simulink library "commanabbnd2"  (Simulink 5.0)
values from neighbouring files (symbols this model uses):
  i = i + 1    (= 3)    [eyediasi2.m]
undefined symbols (not defined in the file or in its folder): den, num
libraries: dspsigattribs x20, commanabbnd2 x3, comminteg2 x3
settings Model: RequirementInfo=9  CovMetricSettings=d  Creator=tdelve  LastModifiedBy=mmclerno

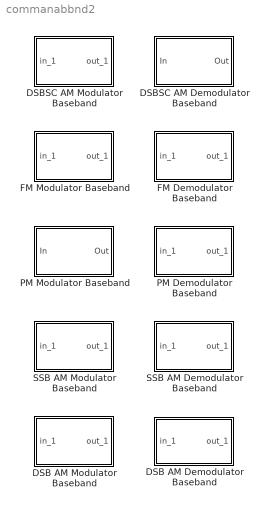
== system commanabbnd2 ==
  DSB AM Demodulator Baseband : Subsystem  mask(DSB AM Demodulator Baseband){Offset=1, num=[4.57 9.14 4.57]*.01, den=[1 -1.3108 .4936], Ph=0, ts=0.001}
      mask prompts: Offset "Output signal offset:"; num "Lowpass filter numerator:"; den "Lowpass filter denominator:"; Ph "Initial phase (rad):"; ts "Sample time (s):"
      mask help: Demodulate the complex envelope of a double-sideband amplitude modulated signal. The input signal must be a sample-based scalar.The output is a 1-D scalar.
      mask init:
      | if ((length(Ph)~=1) | (length(Offset)~=1) | (length(ts)~=1))error('Mask parameters must be scalar values.');end;
      mask Help: helpview(commbhelp)
      mask Display:
      | plot(0,0,100,100,[5+4.5*[0:.15:10] 50 50 50 50+4.5*[0:10]],[85+10*[sin([0:.15:10]*pi*2+cumsum(sin([0:.15:10]*pi/5))/2)] 85 99 75   10*sin([0:10]*pi/5)+85]);
      | disp('DSB AM')
  DSB AM Modulator Baseband : Subsystem  mask(DSB AM Modulator Baseband){Offset=1, Ph=0}
      mask prompts: Offset "Input signal offset:"; Ph "Initial phase (rad):"
      mask help: Output complex envelope of a double-sideband amplitude modulated signal. The input signal must be a sample-based scalar. The output is a 1-D scalar.
      mask init:
      | if ((length(Ph)~=1) | (length(Offset)~=1))error('Mask parameters must be scalar values.');end;
      mask Help: helpview(commbhelp)
      mask Display:
      | plot(0,0,100,100,[4.5*[0:10]+5 50 50 50 50+4.5*[0:.15:10]],[10*sin([0:10]*pi/5)+85 85 99 75 85+10*[sin([0:.15:10]*pi*2+cumsum(sin([0:.15:10]*pi/5))/2)]]);
      | disp('DSB AM')
  DSBSC AM Demodulator Baseband : Subsystem  mask(DSBSC AM Demodulator Baseband){num=[4.57 9.14 4.57]*.01, den=[1 -1.3108 .4936], Ph=pi/2, ts=0.001}
      mask prompts: num "Lowpass filter numerator:"; den "Lowpass filter denominator:"; Ph "Initial phase (rad):"; ts "Sample time (s):"
      mask help: Demodulate the complex envelope of a double-sideband suppressed carrier amplitude modulated signal. The input signal must be a sample-based scalar. The output is a 1-D scalar.
      mask init:
      | if ((length(Ph)~=1) | (length(ts)~=1))error('Mask parameters must be scalar values.');end;
      | pi2=pi*2;
      mask Help: helpview(commbhelp)
      mask Display:
      | plot(0,0,100,100,[5+4.5*[0:.15:10] 50 50 50 50+4.5*[0:10]],[85+10*[sin([0:.15:10]*pi*2+cumsum(sin([0:.15:10]*pi/5))/2)] 85 99 75   10*sin([0:10]*pi/5)+85]);
      | disp('DSBSC AM')
  DSBSC AM Modulator Baseband : Subsystem  mask(DSBSC AM Modulator Baseband){Ph=pi/2}
      mask prompts: Ph "Initial phase (rad):"
      mask help: Output the complex envelope of a double-sideband suppressed carrier amplitude modulated signal. The input signal must be a sample-based scalar. The output is a 1-D scalar.
      mask init:
      | if (length(Ph)~=1) error('Mask parameters must be scalar values.');end;
      | x1=cos(Ph);x2=sin(Ph);pi2=2*pi;
      mask Help: helpview(commbhelp)
      mask Display:
      | plot(0,0,100,100,[4.5*[0:10]+5 50 50 50 50+4.5*[0:.15:10]],[10*sin([0:10]*pi/5)+85 85 99 75 85+10*[sin([0:.15:10]*pi*2+cumsum(sin([0:.15:10]*pi/5))/2)]]);
      | disp('DSBSC AM')
  FM Demodulator Baseband : Subsystem  mask(FM Demodulator Baseband){Ph=0, HzPerVolt=1, num=[4.57 9.14 4.57]*.01, den=[1 -1.3108 .4936], ts=0.001}
      mask prompts: Ph "Initial phase (rad):"; HzPerVolt "Modulation constant (Hertz per volt):"; num "Lowpass filter numerator:"; den "Lowpass filter denominator:"; ts "Sample time (s):"
      mask help: Demodulate the complex envelope of a frequency-modulated signal. The input signal must be a sample-based scalar. The output is a 1-D scalar.
      mask init:
      | if ((length(Ph)~=1) | (length(HzPerVolt)~=1) | (length(ts)~=1))error('Mask parameters must be scalar values.');end;
      | pi2=2*pi;
      | Kc=2*pi*HzPerVolt;
      mask Help: helpview(commbhelp)
      mask Display:
      | plot(0,0,100,100,[5+4.5*[0:.15:10] 50 50 50 50+4.5*[0:10]],[85+10*[sin([0:.15:10]*pi*2+cumsum(sin([0:.15:10]*pi/5))/2)] 85 99 75   10*sin([0:10]*pi/5)+85]);
      | disp('FM')
  FM Modulator Baseband : Subsystem  mask(FM Modulator Baseband){Ph=0, HzPerV=1, ts=0.001, td=Inf}
      mask prompts: Ph "Initial phase (rad):"; HzPerV "Modulation constant (Hertz per volt):"; ts "Sample time (s):"; td "Symbol interval (s):"
      mask help: Output complex baseband signal frequency-modulated by the input signal. For digital modulation, set the Symbol Interval parameter to the desired symbol. For analog modulation, set the Symbol Interval parameter to Inf. The input signal must be a sample-based scalar. The output is a 1-D scalar.
      mask init:
      | if ((length(Ph)~=1) | (length(HzPerV)~=1) | (length(ts)~=1) | (length(td)~=1))error('Mask parameters must be scalar values.');end;
      | Kc =2*pi*HzPerV;if isinf(td),td=realmax;end;
      mask Help: helpview(commbhelp)
      mask Display:
      | plot(0,0,100,100,[4.5*[0:10]+5 50 50 50 50+4.5*[0:.15:10]],[10*sin([0:10]*pi/5)+85 85 99 75 85+10*[sin([0:.15:10]*pi*2+cumsum(sin([0:.15:10]*pi/5))/2)]]);
      | disp('FM')
  PM Demodulator Baseband : Subsystem  mask(PM Demodulator Baseband){Ph=0, Kc=1, num=[4.57 9.14 4.57]*.01, den=[1 -1.3108 .4936], HzPerVolt=1, ts=0.001}
      mask prompts: Ph "Initial phase (rad):"; Kc "Modulation constant (Radians per volt):"; num "Lowpass filter numerator:"; den "Lowpass filter denominator:"; HzPerVolt "VCO gain (Hertz per volt):"; ts "Sample time (s):"
      mask help: Demodulate the complex envelope of a phase-modulated signal. The input signal must be a sample-based scalar. The output is a 1-D scalar.
      mask init:
      | if ((length(Ph)~=1) | (length(HzPerVolt)~=1) | (length(ts)~=1) | (length(Kc)~=1))error('Mask parameters must be scalar values.');end;
      | Kv=2*pi*HzPerVolt;
      mask Help: helpview(commbhelp)
      mask Display:
      | plot(0,0,100,100,[5+4.5*[0:.15:10] 50 50 50 50+4.5*[0:10]],[85+10*[sin([0:.15:10]*pi*2+cumsum(sin([0:.15:10]*pi/5))/2)] 85 99 75   10*sin([0:10]*pi/5)+85]);
      | disp('PM')
  PM Modulator Baseband : Subsystem  mask(PM Modulator Baseband){Ph=0, Kc=1}
      mask prompts: Ph "Initial phase (rad):"; Kc "Modulation constant (Radians per volt):"
      mask help: Output the complex envelope of a phase-modulated signal. The input signal must be a sample-based scalar. The output is a 1-D scalar.
      mask init:
      | if ((length(Ph)~=1) | (length(Kc)~=1))error('Mask parameters must be scalar values.');end;
      mask Help: helpview(commbhelp)
      mask Display:
      | plot(0,0,100,100,[4.5*[0:10]+5 50 50 50 50+4.5*[0:.15:10]],[10*sin([0:10]*pi/5)+85 85 99 75 85+10*[sin([0:.15:10]*pi*2+cumsum(sin([0:.15:10]*pi/5))/2)]]);
      | disp('PM')
  SSB AM Demodulator Baseband : Subsystem  mask(SSB AM Demodulator Baseband){num=[4.57 9.14 4.57]*.01, den=[1 -1.3108 .4936], Ph=0, ts=0.001}
      mask prompts: num "Lowpass filter numerator:"; den "Lowpass filter denominator:"; Ph "Initial phase (rad):"; ts "Sample time (s):"
      mask help: Demodulate the complex envelope of a single-sideband amplitude modulated signal. The input signal must be a sample-based scalar. The output is a 1-D scalar.
      mask init:
      | if ((length(Ph)~=1) | (length(ts)~=1))error('Mask parameters must be scalar values.');end;
      | x1=cos(-Ph);x2=sin(-Ph);
      mask Help: helpview(commbhelp)
      mask Display:
      | plot(0,0,100,100,[5+4.5*[0:.15:10] 50 50 50 50+4.5*[0:10]],[85+10*[sin([0:.15:10]*pi*2+cumsum(sin([0:.15:10]*pi/5))/2)] 85 99 75   10*sin([0:10]*pi/5)+85]);
      | disp('SSB AM')
  SSB AM Modulator Baseband : Subsystem  mask(SSB AM Modulator Baseband){Ph=0, ban=10, dly=0.01, ts=0.001, sd=upper}
      mask prompts: Ph "Initial phase (rad):"; ban "Bandwidth of the input signal (Hz):"; dly "Time delay for Hilbert transform filter (s):"; ts "Sample time (s):"; sd "Sideband to modulate:"
      mask help: Output complex envelope of a single-sideband amplitude modulated signal. The input signal must be a sample-based scalar. The output is a 1-D scalar.
      mask init:
      | if ((length(Ph)~=1) | (length(ban)~=1) | (length(ts)~=1) | (length(dly)~=1))error('Mask parameters must be scalar values.');end;
      | if dly/ts<3 error('Time delay is too small compared to the Sample time value');end;
      | if ban>1/ts, ban=1/ts-ts;end;if(dly/ts>1000)
      | error(['The filter coefficients will take too long to compute.'...
      |         'Try reducing the length of the impulse response by increasing the sample time, or decreasing the delay'])
      | else
      | [num,den]=hilbiir(ts,dly,ban);pi2=2*pi;pih=pi/2;
      | k=-1;if lower(sd)=='lower',k=1;end;
      | end;
      mask Help: helpview(commbhelp)
      mask StyleString: edit,edit,edit,edit,popup(Upper|Lower)
      mask Display:
      | plot(0,0,100,100,[4.5*[0:10]+5 50 50 50 50+4.5*[0:.15:10]],[10*sin([0:10]*pi/5)+85 85 99 75 85+10*[sin([0:.15:10]*pi*2+cumsum(sin([0:.15:10]*pi/5))/2)]]);
      | disp('SSB AM')

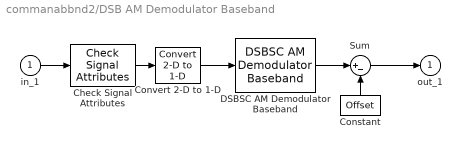
== system commanabbnd2/DSB AM Demodulator Baseband ==
  in_1 : Inport
  Check Signal Attributes : dspsigattribs/Check Signal Attributes  SigAttribCheckMethod=Does not match attributes exactly  Complexity=Ignore  Frame=Sample-based  DimsCheckMethod=Is...  Dimensions=Scalar (1-D or 2-D)  DatatypeCheckMethod=Ignore  DatatypeGeneral=Boolean  DtypeFloatSpecific=Any floating-point  DtypeFixedSpecific=Any fixed-point  DtypeIntSpecific=Any integer  SampleMode=Ignore
  Constant : Constant  Orientation=up  Value=Offset
  Convert 2-D to 1-D : dspsigattribs/Convert 2-D to 1-D
  DSBSC AM Demodulator Baseband : commanabbnd2/DSBSC AM Demodulator Baseband  num=num  den=den  Ph=Ph  ts=ts
  Sum : Sum  Inputs=|+-  SaturateOnIntegerOverflow=on  InputSameDT=on
  out_1 : Outport  InitialOutput=0
  wires:
  DSBSC AM Demodulator Baseband/1 -> Sum/1
  in_1/1 -> Check Signal Attributes/1
  Constant/1 -> Sum/2
  Sum/1 -> out_1/1
  Convert 2-D to 1-D/1 -> DSBSC AM Demodulator Baseband/1
  Check Signal Attributes/1 -> Convert 2-D to 1-D/1

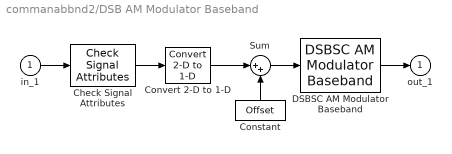
== system commanabbnd2/DSB AM Modulator Baseband ==
  in_1 : Inport
  Check Signal Attributes : dspsigattribs/Check Signal Attributes  SigAttribCheckMethod=Does not match attributes exactly  Complexity=Ignore  Frame=Sample-based  DimsCheckMethod=Is...  Dimensions=Scalar (1-D or 2-D)  DatatypeCheckMethod=Ignore  DatatypeGeneral=Boolean  DtypeFloatSpecific=Any floating-point  DtypeFixedSpecific=Any fixed-point  DtypeIntSpecific=Any integer  SampleMode=Ignore
  Constant : Constant  Orientation=up  Value=Offset
  Convert 2-D to 1-D : dspsigattribs/Convert 2-D to 1-D
  DSBSC AM Modulator Baseband : commanabbnd2/DSBSC AM Modulator Baseband  Ph=Ph
  Sum : Sum  Inputs=|++  SaturateOnIntegerOverflow=on  InputSameDT=on
  out_1 : Outport  InitialOutput=0
  wires:
  Constant/1 -> Sum/2
  in_1/1 -> Check Signal Attributes/1
  Sum/1 -> DSBSC AM Modulator Baseband/1
  DSBSC AM Modulator Baseband/1 -> out_1/1
  Convert 2-D to 1-D/1 -> Sum/1
  Check Signal Attributes/1 -> Convert 2-D to 1-D/1

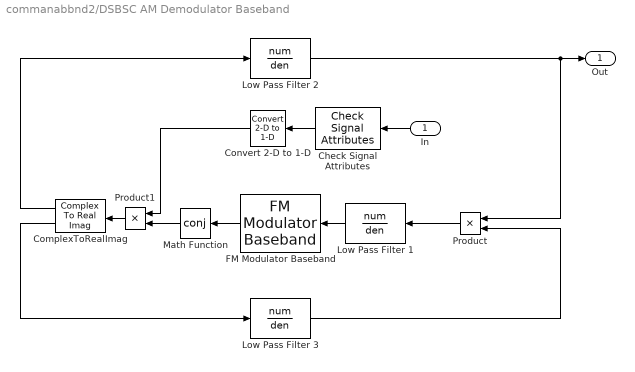
== system commanabbnd2/DSBSC AM Demodulator Baseband ==
  In : Inport  Orientation=left
  Check Signal Attributes : dspsigattribs/Check Signal Attributes  Orientation=left  SigAttribCheckMethod=Does not match attributes exactly  Complexity=Ignore  Frame=Sample-based  DimsCheckMethod=Is...  Dimensions=Scalar (1-D or 2-D)  DatatypeCheckMethod=Ignore  DatatypeGeneral=Boolean  DtypeFloatSpecific=Any floating-point  DtypeFixedSpecific=Any fixed-point  DtypeIntSpecific=Any integer  SampleMode=Ignore
  ComplexToRealImag : ComplexToRealImag  Orientation=left
  Convert 2-D to 1-D : dspsigattribs/Convert 2-D to 1-D  Orientation=left
  FM Modulator Baseband : commanabbnd2/FM Modulator Baseband  Orientation=left  Ph=Ph  HzPerV=1  ts=ts  td=Inf
  Low Pass Filter 1 : DiscreteFilter  Orientation=left  Numerator=num  Denominator=den  SampleTime=ts
  Low Pass Filter 2 : DiscreteFilter  Numerator=num  Denominator=den  SampleTime=ts
  Low Pass Filter 3 : DiscreteFilter  Numerator=num  Denominator=den  SampleTime=ts
  Math Function : Math  Orientation=left  Operator=conj
  Product : Product  Orientation=left  SaturateOnIntegerOverflow=on  InputSameDT=on
  Product1 : Product  Orientation=left  SaturateOnIntegerOverflow=on  InputSameDT=on
  Out : Outport  InitialOutput=0
  wires:
  ComplexToRealImag/1 -> Low Pass Filter 2/1
  ComplexToRealImag/2 -> Low Pass Filter 3/1
  Product/1 -> Low Pass Filter 1/1
  Product1/1 -> ComplexToRealImag/1
  In/1 -> Check Signal Attributes/1
  Math Function/1 -> Product1/2
  FM Modulator Baseband/1 -> Math Function/1
  Low Pass Filter 3/1 -> Product/2
  Low Pass Filter 1/1 -> FM Modulator Baseband/1
  Low Pass Filter 2/1 -> Product/1, Out/1
  Convert 2-D to 1-D/1 -> Product1/1
  Check Signal Attributes/1 -> Convert 2-D to 1-D/1

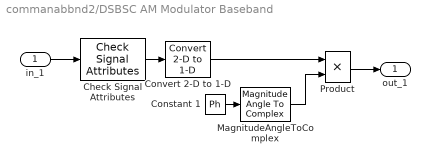
== system commanabbnd2/DSBSC AM Modulator Baseband ==
  in_1 : Inport
  Check Signal Attributes : dspsigattribs/Check Signal Attributes  SigAttribCheckMethod=Does not match attributes exactly  Complexity=Ignore  Frame=Sample-based  DimsCheckMethod=Is...  Dimensions=Scalar (1-D or 2-D)  DatatypeCheckMethod=Ignore  DatatypeGeneral=Boolean  DtypeFloatSpecific=Any floating-point  DtypeFixedSpecific=Any fixed-point  DtypeIntSpecific=Any integer  SampleMode=Ignore
  Constant 1 : Constant  Value=Ph
  Convert 2-D to 1-D : dspsigattribs/Convert 2-D to 1-D
  MagnitudeAngleToComplex : MagnitudeAngleToComplex  Input=Angle  ConstantPart=1
  Product : Product  SaturateOnIntegerOverflow=on  InputSameDT=on
  out_1 : Outport  InitialOutput=0
  wires:
  in_1/1 -> Check Signal Attributes/1
  MagnitudeAngleToComplex/1 -> Product/2
  Constant 1/1 -> MagnitudeAngleToComplex/1
  Product/1 -> out_1/1
  Convert 2-D to 1-D/1 -> Product/1
  Check Signal Attributes/1 -> Convert 2-D to 1-D/1

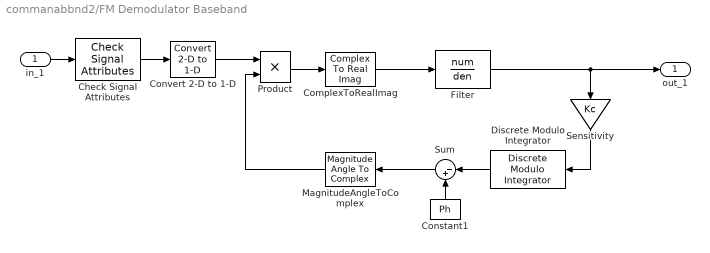
== system commanabbnd2/FM Demodulator Baseband ==
  in_1 : Inport
  Check Signal Attributes : dspsigattribs/Check Signal Attributes  SigAttribCheckMethod=Does not match attributes exactly  Complexity=Ignore  Frame=Sample-based  DimsCheckMethod=Is...  Dimensions=Scalar (1-D or 2-D)  DatatypeCheckMethod=Ignore  DatatypeGeneral=Boolean  DtypeFloatSpecific=Any floating-point  DtypeFixedSpecific=Any fixed-point  DtypeIntSpecific=Any integer  SampleMode=Ignore
  ComplexToRealImag : ComplexToRealImag  Output=Imag
  Constant1 : Constant  Orientation=up  Value=Ph
  Convert 2-D to 1-D : dspsigattribs/Convert 2-D to 1-D
  Discrete Modulo Integrator : comminteg2/Discrete Modulo Integrator  Orientation=left  modu=pi2  init=0  ts=ts
  Filter : DiscreteFilter  Numerator=num  Denominator=den  SampleTime=ts
  MagnitudeAngleToComplex : MagnitudeAngleToComplex  Orientation=left  Input=Angle  ConstantPart=1
  Product : Product  SaturateOnIntegerOverflow=on  InputSameDT=on
  Sensitivity : Gain  Orientation=down  Gain=Kc  SaturateOnIntegerOverflow=on
  Sum : Sum  Orientation=left  Inputs=|-+  SaturateOnIntegerOverflow=on  InputSameDT=on
  out_1 : Outport  InitialOutput=0
  wires:
  Filter/1 -> Sensitivity/1, out_1/1
  in_1/1 -> Check Signal Attributes/1
  Product/1 -> ComplexToRealImag/1
  ComplexToRealImag/1 -> Filter/1
  MagnitudeAngleToComplex/1 -> Product/2
  Sensitivity/1 -> Discrete Modulo Integrator/1
  Discrete Modulo Integrator/1 -> Sum/1
  Constant1/1 -> Sum/2
  Sum/1 -> MagnitudeAngleToComplex/1
  Convert 2-D to 1-D/1 -> Product/1
  Check Signal Attributes/1 -> Convert 2-D to 1-D/1

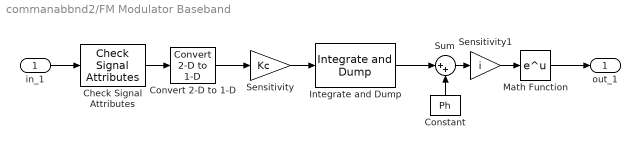
== system commanabbnd2/FM Modulator Baseband ==
  in_1 : Inport
  Check Signal Attributes : dspsigattribs/Check Signal Attributes  SigAttribCheckMethod=Does not match attributes exactly  Complexity=Ignore  Frame=Sample-based  DimsCheckMethod=Is...  Dimensions=Scalar (1-D or 2-D)  DatatypeCheckMethod=Ignore  DatatypeGeneral=Boolean  DtypeFloatSpecific=Any floating-point  DtypeFixedSpecific=Any fixed-point  DtypeIntSpecific=Any integer  SampleMode=Ignore
  Constant : Constant  Orientation=up  Value=Ph
  Convert 2-D to 1-D : dspsigattribs/Convert 2-D to 1-D
  Integrate and Dump : comminteg2/Integrate and Dump  limit=2*pi  td=td  ts=ts
  Math Function : Math
  Sensitivity : Gain  Gain=Kc  SaturateOnIntegerOverflow=on
  Sensitivity1 : Gain  Gain=i  SaturateOnIntegerOverflow=on
  Sum : Sum  Inputs=|++  SaturateOnIntegerOverflow=on  InputSameDT=on
  out_1 : Outport  InitialOutput=0
  wires:
  Sensitivity/1 -> Integrate and Dump/1
  in_1/1 -> Check Signal Attributes/1
  Integrate and Dump/1 -> Sum/1
  Constant/1 -> Sum/2
  Sum/1 -> Sensitivity1/1
  Sensitivity1/1 -> Math Function/1
  Math Function/1 -> out_1/1
  Convert 2-D to 1-D/1 -> Sensitivity/1
  Check Signal Attributes/1 -> Convert 2-D to 1-D/1

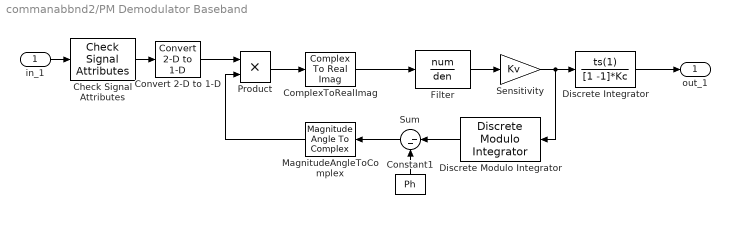
== system commanabbnd2/PM Demodulator Baseband ==
  in_1 : Inport
  Check Signal Attributes : dspsigattribs/Check Signal Attributes  SigAttribCheckMethod=Does not match attributes exactly  Complexity=Ignore  Frame=Sample-based  DimsCheckMethod=Is...  Dimensions=Scalar (1-D or 2-D)  DatatypeCheckMethod=Ignore  DatatypeGeneral=Boolean  DtypeFloatSpecific=Any floating-point  DtypeFixedSpecific=Any fixed-point  DtypeIntSpecific=Any integer  SampleMode=Ignore
  ComplexToRealImag : ComplexToRealImag  Output=Imag
  Constant1 : Constant  Orientation=up  Value=Ph
  Convert 2-D to 1-D : dspsigattribs/Convert 2-D to 1-D
  Discrete Integrator : DiscreteFilter  Numerator=ts(1)  Denominator=[1 -1]*Kc  SampleTime=ts
  Discrete Modulo Integrator : comminteg2/Discrete Modulo Integrator  Orientation=left  modu=2*pi  init=0  ts=ts
  Filter : DiscreteFilter  Numerator=num  Denominator=den  SampleTime=ts
  MagnitudeAngleToComplex : MagnitudeAngleToComplex  Orientation=left  Input=Angle  ConstantPart=1
  Product : Product  SaturateOnIntegerOverflow=on  InputSameDT=on
  Sensitivity : Gain  Gain=Kv  SaturateOnIntegerOverflow=on
  Sum : Sum  Orientation=left  Inputs=|--  SaturateOnIntegerOverflow=on  InputSameDT=on
  out_1 : Outport  InitialOutput=0
  wires:
  Sum/1 -> MagnitudeAngleToComplex/1
  Constant1/1 -> Sum/2
  Discrete Modulo Integrator/1 -> Sum/1
  MagnitudeAngleToComplex/1 -> Product/2
  ComplexToRealImag/1 -> Filter/1
  Product/1 -> ComplexToRealImag/1
  in_1/1 -> Check Signal Attributes/1
  Filter/1 -> Sensitivity/1
  Sensitivity/1 -> Discrete Integrator/1, Discrete Modulo Integrator/1
  Discrete Integrator/1 -> out_1/1
  Convert 2-D to 1-D/1 -> Product/1
  Check Signal Attributes/1 -> Convert 2-D to 1-D/1

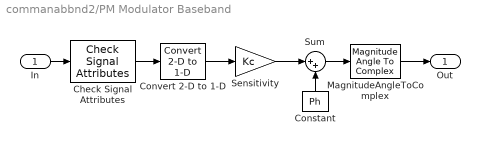
== system commanabbnd2/PM Modulator Baseband ==
  In : Inport
  Check Signal Attributes : dspsigattribs/Check Signal Attributes  SigAttribCheckMethod=Does not match attributes exactly  Complexity=Ignore  Frame=Sample-based  DimsCheckMethod=Is...  Dimensions=Scalar (1-D or 2-D)  DatatypeCheckMethod=Ignore  DatatypeGeneral=Boolean  DtypeFloatSpecific=Any floating-point  DtypeFixedSpecific=Any fixed-point  DtypeIntSpecific=Any integer  SampleMode=Ignore
  Constant : Constant  Orientation=up  Value=Ph
  Convert 2-D to 1-D : dspsigattribs/Convert 2-D to 1-D
  MagnitudeAngleToComplex : MagnitudeAngleToComplex  Input=Angle  ConstantPart=1
  Sensitivity : Gain  Gain=Kc  SaturateOnIntegerOverflow=on
  Sum : Sum  Inputs=|++  SaturateOnIntegerOverflow=on  InputSameDT=on
  Out : Outport  InitialOutput=0
  wires:
  In/1 -> Check Signal Attributes/1
  Constant/1 -> Sum/2
  Sum/1 -> MagnitudeAngleToComplex/1
  Sensitivity/1 -> Sum/1
  MagnitudeAngleToComplex/1 -> Out/1
  Convert 2-D to 1-D/1 -> Sensitivity/1
  Check Signal Attributes/1 -> Convert 2-D to 1-D/1

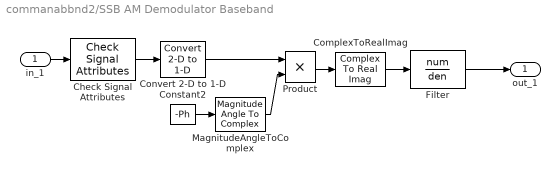
== system commanabbnd2/SSB AM Demodulator Baseband ==
  in_1 : Inport
  Check Signal Attributes : dspsigattribs/Check Signal Attributes  SigAttribCheckMethod=Does not match attributes exactly  Complexity=Ignore  Frame=Sample-based  DimsCheckMethod=Is...  Dimensions=Scalar (1-D or 2-D)  DatatypeCheckMethod=Ignore  DatatypeGeneral=Boolean  DtypeFloatSpecific=Any floating-point  DtypeFixedSpecific=Any fixed-point  DtypeIntSpecific=Any integer  SampleMode=Ignore
  ComplexToRealImag : ComplexToRealImag  Output=Real
  Constant2 : Constant  Value=-Ph
  Convert 2-D to 1-D : dspsigattribs/Convert 2-D to 1-D
  Filter : DiscreteFilter  Numerator=num  Denominator=den  SampleTime=ts
  MagnitudeAngleToComplex : MagnitudeAngleToComplex  Input=Angle  ConstantPart=1
  Product : Product  SaturateOnIntegerOverflow=on  InputSameDT=on
  out_1 : Outport  InitialOutput=0
  wires:
  MagnitudeAngleToComplex/1 -> Product/2
  Constant2/1 -> MagnitudeAngleToComplex/1
  in_1/1 -> Check Signal Attributes/1
  Product/1 -> ComplexToRealImag/1
  ComplexToRealImag/1 -> Filter/1
  Filter/1 -> out_1/1
  Convert 2-D to 1-D/1 -> Product/1
  Check Signal Attributes/1 -> Convert 2-D to 1-D/1

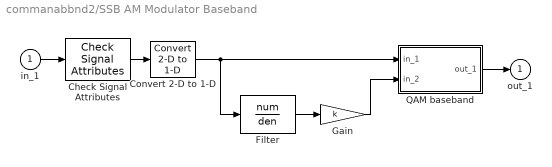
== system commanabbnd2/SSB AM Modulator Baseband ==
  in_1 : Inport
  Check Signal Attributes : dspsigattribs/Check Signal Attributes  SigAttribCheckMethod=Does not match attributes exactly  Complexity=Ignore  Frame=Sample-based  DimsCheckMethod=Is...  Dimensions=Scalar (1-D or 2-D)  DatatypeCheckMethod=Ignore  DatatypeGeneral=Boolean  DtypeFloatSpecific=Any floating-point  DtypeFixedSpecific=Any fixed-point  DtypeIntSpecific=Any integer  SampleMode=Ignore
  Convert 2-D to 1-D : dspsigattribs/Convert 2-D to 1-D
  Filter : DiscreteFilter  Numerator=num  Denominator=den  SampleTime=ts
  Gain : Gain  Gain=k  SaturateOnIntegerOverflow=on
  QAM baseband : Subsystem  mask(QAM Baseband){Ph=Ph}
      mask prompts: Ph "Initial phase (rad):"
      mask help: Modulate the in-phase and quadrature component signal from the 1st and 2nd input ports, baseband simulation.
      mask Help: helpview(commbhelp)
      mask Display:
      | plot(0,0,100,100,[4.5*[0:10]+5 50 50 50 50+4.5*[0:.3:10]],[10*sin([0:10]*pi/5)+85 85 99 75 85+10*[sin([0:.3:10]*pi/5).*sin([0:.3:10]*pi*2)]]);
      | disp('QAM')
  out_1 : Outport  InitialOutput=0
  wires:
  Gain/1 -> QAM baseband/2(in_2)
  Filter/1 -> Gain/1
  in_1/1 -> Check Signal Attributes/1
  QAM baseband/1(out_1) -> out_1/1
  Convert 2-D to 1-D/1 -> QAM baseband/1(in_1), Filter/1
  Check Signal Attributes/1 -> Convert 2-D to 1-D/1

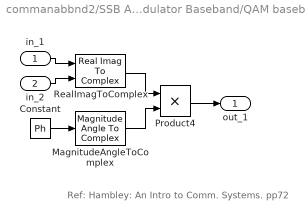
== system commanabbnd2/SSB AM Modulator Baseband/QAM baseband ==
  note: Ref: Hambley: An Intro to Comm. Systems. pp72
  in_1 : Inport
  in_2 : Inport  Port=2
  Constant : Constant  Value=Ph
  MagnitudeAngleToComplex : MagnitudeAngleToComplex  Input=Angle  ConstantPart=1
  Product4 : Product  SaturateOnIntegerOverflow=on  InputSameDT=on
  RealImagToComplex : RealImagToComplex
  out_1 : Outport  InitialOutput=0
  wires:
  MagnitudeAngleToComplex/1 -> Product4/2
  Constant/1 -> MagnitudeAngleToComplex/1
  RealImagToComplex/1 -> Product4/1
  in_2/1 -> RealImagToComplex/2
  in_1/1 -> RealImagToComplex/1
  Product4/1 -> out_1/1
